simulink model "mass_spring_damper_simulink_project_solution"  (R2022a)
settings: Solver=ode45  StartTime=0.0  StopTime=Sim_Time  MaxStep=0.01  RelTol=1e-3  EnableMultiTasking=on
undefined symbols (not defined in the file): b1, b2, F, k1, k2, M1, M2
settings Model: Creator=dzr3qn  LastModifiedBy=Dr. Ryan Aly
settings SolverCC: AlgebraicLoopSolver=TrustRegion
settings DataIOCC: LimitDataPoints=on  SaveFormat=Array  ReturnWorkspaceOutputs=off
settings OptimizationCC: LifeSpan=inf
settings DebuggingCC: SolverPrmCheckMsg=warning  UnconnectedInputMsg=warning  UnconnectedOutputMsg=warning  UnconnectedLineMsg=warning  SFUnexpectedBacktrackingDiag=warning  SFNoUnconditionalDefaultTransitionDiag=warning  SFExecutionAtInitializationDiag=none  SFMachineParentedDataDiag=warning  ArithmeticOperatorsInVariantConditions=warning
settings HardwareCC: ProdBitPerPointer=32  ProdBitPerSizeT=32  ProdBitPerPtrDiffT=32  ProdLargestAtomicFloat=None  ProdIntDivRoundTo=Undefined  ProdEndianess=Unspecified  ProdWordSize=32  ProdHWDeviceType=32-bit Generic
settings ModelReferenceCC: PropagateSignalLabelsOutOfModel=off
settings SFSimCC: SimUseLocalCustomCode=off  CustomCodeUndefinedFunction=UseInterfaceOnly
settings RTWCC: RTWUseLocalCustomCode=off
settings CodeAppCC: StateflowObjectComments=on
settings GRTTargetCC: TargetLangStandard=C89/C90 (ANSI)
settings ConfigComp: CovMetricSettings=dw  CovSaveCumulativeToWorkspaceVar=on  CovSaveSingleToWorkspaceVar=on  CovExternalEMLEnable=off  CovSFcnEnable=off

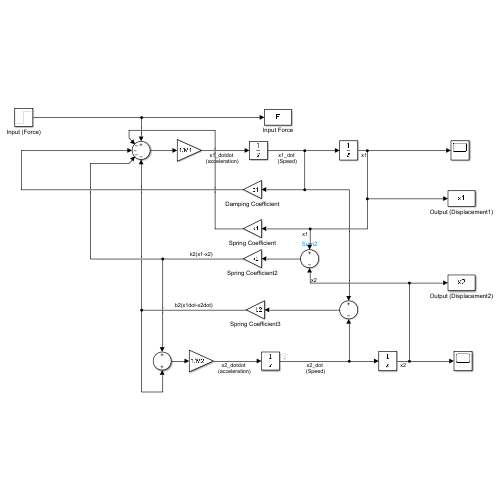
[thumbnail: Simulink's stored preview of the top-level diagram]
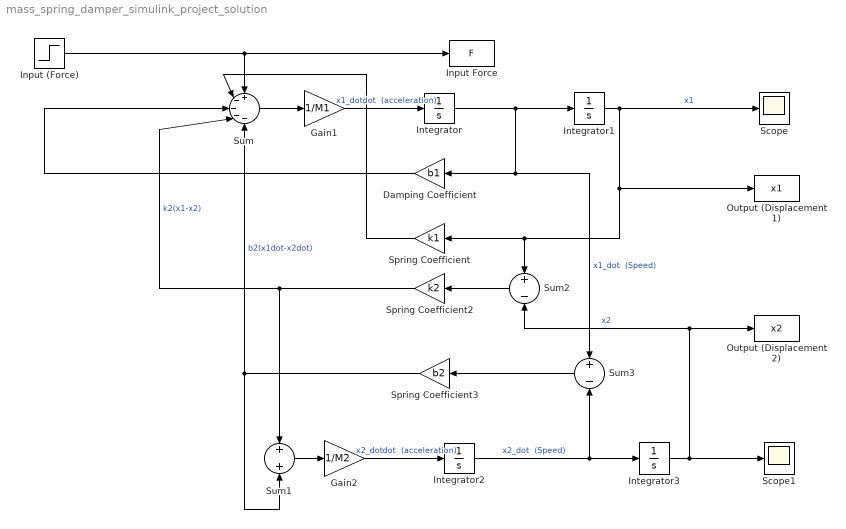
== system mass_spring_damper_simulink_project_solution ==
  Damping Coefficient : Gain  Gain=b1
  Gain1 : Gain  Gain=1/M1
  Gain2 : Gain  Gain=1/M2
  Input (Force) : Step  After=F  SampleTime=0
  Input Force : ToWorkspace  VariableName=F  SaveFormat=Timeseries  SampleTime=-1
  Integrator{,1..3} (4 alike) : Integrator
  Output (Displacement1) : ToWorkspace  VariableName=x1  SaveFormat=Timeseries  SampleTime=-1
  Output (Displacement2) : ToWorkspace  VariableName=x2  SaveFormat=Timeseries  SampleTime=-1
  Scope : Scope
  Scope1 : Scope
  Spring Coefficient : Gain  Gain=k1
  Spring Coefficient2 : Gain  Gain=k2
  Spring Coefficient3 : Gain  Gain=b2
  Sum : Sum  Inputs=+----
  Sum1 : Sum
  Sum2 : Sum  Inputs=+-
  Sum3 : Sum  Inputs=+-
  wires:
  Integrator/1 -> Sum3/1, Damping Coefficient/1, Integrator1/1  "x1_dot  (Speed)"
  Integrator1/1 -> Output (Displacement1)/1, Sum2/1, Spring Coefficient/1, Scope/1  "x1"
  Sum/1 -> Gain1/1
  Gain1/1 -> Integrator/1  "x1_dotdot  (acceleration)"
  Damping Coefficient/1 -> Sum/3
  Spring Coefficient/1 -> Sum/2
  Input (Force)/1 -> Input Force/1, Sum/1
  Gain2/1 -> Integrator2/1  "x2_dotdot  (acceleration)"
  Integrator2/1 -> Sum3/2, Integrator3/1  "x2_dot  (Speed)"
  Sum1/1 -> Gain2/1
  Integrator3/1 -> Scope1/1, Sum2/2, Output (Displacement2)/1  "x2"
  Sum2/1 -> Spring Coefficient2/1
  Spring Coefficient2/1 -> Sum/4, Sum1/1  "k2(x1-x2)"
  Sum3/1 -> Spring Coefficient3/1
  Spring Coefficient3/1 -> Sum1/2, Sum/5  "b2(x1dot-x2dot)"
